simulink model "blockdemo"  (Simulink 6.3)
settings: Solver=VariableStepDiscrete  StartTime=0.0  StopTime=500  RelTol=1e-3
InitFcn:
  | %% DSPBuilder Start
  | alt_dspbuilder_update_model(bdroot)
  | %% DSPBuilder End
libraries: allblocks_alteradspbuilder2 x16, simulink x2
settings Model: Creator=cpurcell  LastModifiedBy=delphick
settings DebuggingCC: MultiTaskDSMMsg=error

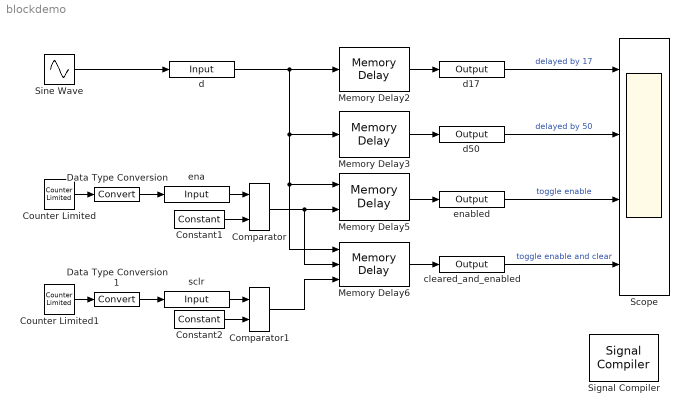
== system blockdemo ==
  Comparator : allblocks_alteradspbuilder2/Comparator  direction=a == b
  Comparator1 : allblocks_alteradspbuilder2/Comparator  direction=a == b
  Constant1 : allblocks_alteradspbuilder2/Constant  mask_cst=1  BusType=Unsigned Integer  bwl=1  bwr=0  SpecifyClock=off  clock=default_clock
  Constant2 : allblocks_alteradspbuilder2/Constant  mask_cst=10  BusType=Unsigned Integer  bwl=8  bwr=0  SpecifyClock=off  clock=default_clock
  Counter Limited : simulink/Sources/Counter Limited  uplimit=2  tsamp=1
      settings: AttributesFormatString=limit = %<uplimit>
  Counter Limited1 : simulink/Sources/Counter Limited  uplimit=31  tsamp=1
      settings: AttributesFormatString=limit = %<uplimit>
  Data Type Conversion : DataTypeConversion
  Data Type Conversion1 : DataTypeConversion
  Memory Delay2 : allblocks_alteradspbuilder2/Memory Delay  BusType=Inferred  bwl=8  bwr=0  pipeline=17  ram_type=M512  use_ena=off  use_sclr=off
  Memory Delay3 : allblocks_alteradspbuilder2/Memory Delay  BusType=Inferred  bwl=8  bwr=0  pipeline=50  ram_type=M512  use_ena=off  use_sclr=off
  Memory Delay5 : allblocks_alteradspbuilder2/Memory Delay  BusType=Inferred  bwl=8  bwr=0  pipeline=2  ram_type=AUTO  use_ena=on  use_sclr=off
  Memory Delay6 : allblocks_alteradspbuilder2/Memory Delay  BusType=Inferred  bwl=8  bwr=0  pipeline=2  ram_type=AUTO  use_ena=on  use_sclr=on
  Scope : Scope  NumInputPorts=4
      settings: TimeRange=500  YMin=-200~-200~-200~-200  YMax=200~200~200~200
  Signal Compiler : allblocks_alteradspbuilder2/Signal Compiler  DeviceFamily=Stratix III  DeviceName=AUTO  EnableSignalTap=off  SignalTapDepth=128  UseBoardBlock=off  StpUseDefaultClock=on  StpClock=clock
  Sine Wave : Sin  SineType=Sample based  Amplitude=127  Frequency=0.25  Samples=100  SampleTime=1
  cleared_and_enabled : allblocks_alteradspbuilder2/Output  iofile=C:\workspace_clean\Documentation\DesignExamples\Tutorials\UnitBlocks\Storage\MemoryDelay\tb_blockdemo\blockdemo_cleared_and_enabled.capture  BusType=Signed Integer  bwl=8  bwr=0  PORTTYPE=Output
  d : allblocks_alteradspbuilder2/Input  iofile=C:\workspace_clean\Documentation\DesignExamples\Tutorials\UnitBlocks\Storage\MemoryDelay\tb_blockdemo\blockdemo_d.salt  BusType=Signed Integer  bwl=8  bwr=0  SpecifyClock=off  clock=default_clock  PORTTYPE=Input
  d17 : allblocks_alteradspbuilder2/Output  iofile=C:\workspace_clean\Documentation\DesignExamples\Tutorials\UnitBlocks\Storage\MemoryDelay\tb_blockdemo\blockdemo_d17.capture  BusType=Signed Integer  bwl=8  bwr=0  PORTTYPE=Output
  d50 : allblocks_alteradspbuilder2/Output  iofile=C:\workspace_clean\Documentation\DesignExamples\Tutorials\UnitBlocks\Storage\MemoryDelay\tb_blockdemo\blockdemo_d50.capture  BusType=Signed Integer  bwl=8  bwr=0  PORTTYPE=Output
  ena : allblocks_alteradspbuilder2/Input  iofile=C:\workspace_clean\Documentation\DesignExamples\Tutorials\UnitBlocks\Storage\MemoryDelay\tb_blockdemo\blockdemo_ena.salt  BusType=Unsigned Integer  bwl=8  bwr=0  SpecifyClock=off  clock=default_clock  PORTTYPE=Input
  enabled : allblocks_alteradspbuilder2/Output  iofile=C:\workspace_clean\Documentation\DesignExamples\Tutorials\UnitBlocks\Storage\MemoryDelay\tb_blockdemo\blockdemo_enabled.capture  BusType=Signed Integer  bwl=8  bwr=0  PORTTYPE=Output
  sclr : allblocks_alteradspbuilder2/Input  iofile=C:\workspace_clean\Documentation\DesignExamples\Tutorials\UnitBlocks\Storage\MemoryDelay\tb_blockdemo\blockdemo_sclr.salt  BusType=Signed Integer  bwl=8  bwr=0  SpecifyClock=off  clock=default_clock  PORTTYPE=Input
  wires:
  Sine Wave/1 -> d/1
  Memory Delay2/1 -> d17/1
  Memory Delay5/1 -> enabled/1
  Counter Limited/1 -> Data Type Conversion/1
  ena/1 -> Comparator/1
  Comparator/1 -> Memory Delay5/2, Memory Delay6/2
  Constant1/1 -> Comparator/2
  d17/1 -> Scope/1  "delayed by 17"
  d/1 -> Memory Delay3/1, Memory Delay5/1, Memory Delay6/1, Memory Delay2/1
  Data Type Conversion/1 -> ena/1
  Memory Delay3/1 -> d50/1
  d50/1 -> Scope/2  "delayed by 50"
  enabled/1 -> Scope/3  "toggle enable"
  Counter Limited1/1 -> Data Type Conversion1/1
  sclr/1 -> Comparator1/1
  Constant2/1 -> Comparator1/2
  Data Type Conversion1/1 -> sclr/1
  Comparator1/1 -> Memory Delay6/3
  cleared_and_enabled/1 -> Scope/4  "toggle enable and clear"
  Memory Delay6/1 -> cleared_and_enabled/1
